simulink model "pwa_sim"  (Simulink 7.4)
settings: Solver=ode23tb  StartTime=0.0  StopTime=SimParam.StopTime  MaxStep=0.05  RelTol=1e-4
values from neighbouring files (symbols this model uses):
  pwactrl = []    [Lyapunov_function.m]
  xcl = pwasys.xcl    [AnsGlblElp.m]    (also in AnsGlblReg.m; AnsPWQElp.m; AnsPWQReg.m; LyapContGeneral.m = zeros(Num_S, 1))
undefined symbols (not defined in the file or in its folder): NonSys, pwaModel, SimParam
settings Model: Creator=Behzad  LastModifiedBy=home
settings OptimizationCC: InitFltsAndDblsToZero=on
settings DebuggingCC: SaveWithParameterizedLinksMsg=none  SignalResolutionControl=TryResolveAllWithWarning  MultiTaskDSMMsg=warning  MultiTaskCondExecSysMsg=none  StrictBusMsg=None
settings RTWCC: IncludeERTFirstTime=on
settings GRTTargetCC: TargetFcnLib=ansi_tfl_tmw.mat

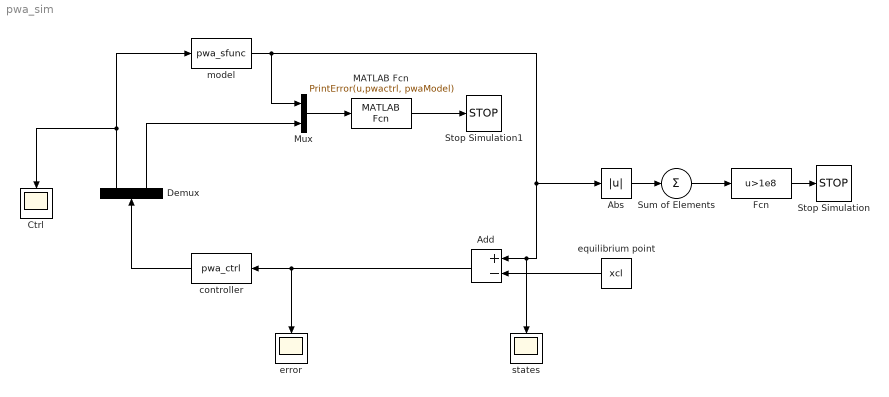
== system pwa_sim ==
  Abs : Abs
  Add : Sum  Inputs=+-  OutDataType=fixdt(1, 16)  OutScaling=2^-10
  Ctrl : Scope
      settings: TickLabels=on  TimeRange=10  YMin=-50  YMax=80  SaveName=sim_ctrl  DataFormat=Array
  Demux : Demux  Outputs=2
  Fcn : Fcn  Expr=u>1e8
  MATLAB Fcn : MATLABFcn  MATLABFcn=PrintError(u,pwactrl, pwaModel)  OutputSignalType=real
  Mux : Mux  Inputs=2
  Stop Simulation : Stop
  Stop Simulation1 : Stop
  Sum of Elements : Sum  Inputs=1  OutDataType=sfix(16)  OutScaling=2^-10
  controller : S-Function  FunctionName=pwa_ctrl  Parameters=pwactrl,SimParam  EnableBusSupport=off
  equilibrium point : Constant  Value=xcl  OutDataType=fixdt(1, 16)  OutScaling=2^0
  error : Scope
      settings: TimeRange=10  YMin=-3.25  YMax=2  SaveName=sim_states  DataFormat=Array
  model : S-Function  FunctionName=pwa_sfunc  Parameters=NonSys,pwaModel,SimParam  EnableBusSupport=off
  states : Scope
      settings: TimeRange=10  YMin=-1.4  YMax=0.4  SaveName=pwa_state
  wires:
  Fcn/1 -> Stop Simulation/1
  Abs/1 -> Sum of Elements/1
  equilibrium point/1 -> Add/2
  Add/1 -> controller/1, error/1
  Sum of Elements/1 -> Fcn/1
  model/1 -> Add/1, states/1, Abs/1, Mux/1
  Demux/1 -> model/1, Ctrl/1
  MATLAB Fcn/1 -> Stop Simulation1/1
  Mux/1 -> MATLAB Fcn/1
  Demux/2 -> Mux/2
  controller/1 -> Demux/1
